simulink model "acc_with_sensor"  (R2021b)
settings: Solver=FixedStepAuto  StartTime=0.0  StopTime=206  FixedStep=0.0005  RelTol=1e-3
InitFcn:
  | G=9.81;
  | m=1660;
  | rw=0.325;
  | Caf=74070;
  | Car=58525;
  | Iz=2778.5;
  | d = 1.502;
  | lf =1.1135;
  | lr =1.5065;
  | L = 2.62;
  | kph2mps=1/3.6;
values from neighbouring files (symbols this model uses):
  Leftdis_PV_switch = 2    [acc_plot_backup.m]
  s_path = [0 1.10508939428 2.2141958029 3.32141571172 4.42705301151 5.53154548532 6.63517443471 7.73808041313 8.84055018688 9.94289959674 11.0453539299 12.1480581097 ... (1001 elements, 1001x1)]    [200_100radius.mat]    (also in LV_Clothoid_S_Turn_path.mat = [0 0.966832089581 1.93621320584 2.90214024471 3.86476766313 ; NEDC_path.mat = [0 0.414605943146 0.832514087334 1.25401518562 1.68216660344; Straight_East_into_curve.mat = [0 1.65770560069 3.32192925577 4.98420060507 6.64484613518 8; acc_plot_backup.m = Station_HV_m)
  X_path = [0 1.10508939428 2.2141958029 3.32141571172 4.42705301151 5.53154548532 6.63517443471 7.73808041313 8.84055018688 9.94289959674 11.0453539299 12.1480581097 ... (1001 elements, 1001x1)]    [200_100radius.mat]    (also in LV_Clothoid_S_Turn_path.mat = [-10 -9.03316791042 -8.06378679416 -7.09785975529 -6.1352323; NEDC_path.mat = [0 0.414605943146 0.832514087334 1.25401518562 1.68216660344; Straight_East_into_curve.mat = [0 1.65770560069 3.32192925577 4.98420060507 6.64484613518 8; acc_plot_backup.m = X_HV_m)
  Y_path = [0 -1.70364610795e-18 -7.41532896709e-18 1.46822109542e-17 4.74557362791e-17 6.12980216762e-17 9.25043977736e-17 1.24088240159e-16 1.5099156923e-16 1.7058517853e-16 1.90629227614e-16 2.09673434424e-16 ... (1001 elements, 1001x1)]    [200_100radius.mat]    (also in LV_Clothoid_S_Turn_path.mat = [0 -8.46153035536e-19 5.07382551045e-18 2.07356032218e-17 3.; NEDC_path.mat = [0 -3.50680326162e-18 -2.14111304971e-18 3.38197671014e-18 3; Straight_East_into_curve.mat = [0 1.29197709199e-18 2.81882429322e-18 3.49020462564e-17 6.7; acc_plot_backup.m = Y_HV_m)
undefined symbols (not defined in the file or in its folder): C_TICK_TIME_S, Cut_in_Secenary_flg, ENUM_ACCSTATE_DISABLED, ENUM_ACCSTATE_OFF, ENUM_ACCSTATE_STANDBY, FALSE, KVDI_ACCLongPressTime_ms, KVDI_ACCMaxActSpeed_kph, KVDI_ACCSetSpdIntial_kph, KVDI_ACCSpdLargeChange_kph, KVDI_LongPressConTime_ms, ONE_FLOAT, ONE_INT, raptor_xcp_function, T, TRUE, UseTTC_switch, ZERO_FLOAT, ZERO_INT
libraries: ADASLibrary x29, simulink x22, Raptor_lib x11, dspstat3 x6, simulink_extras x6, Solver_SF x1, mpclib x1
(part 4 of 9)

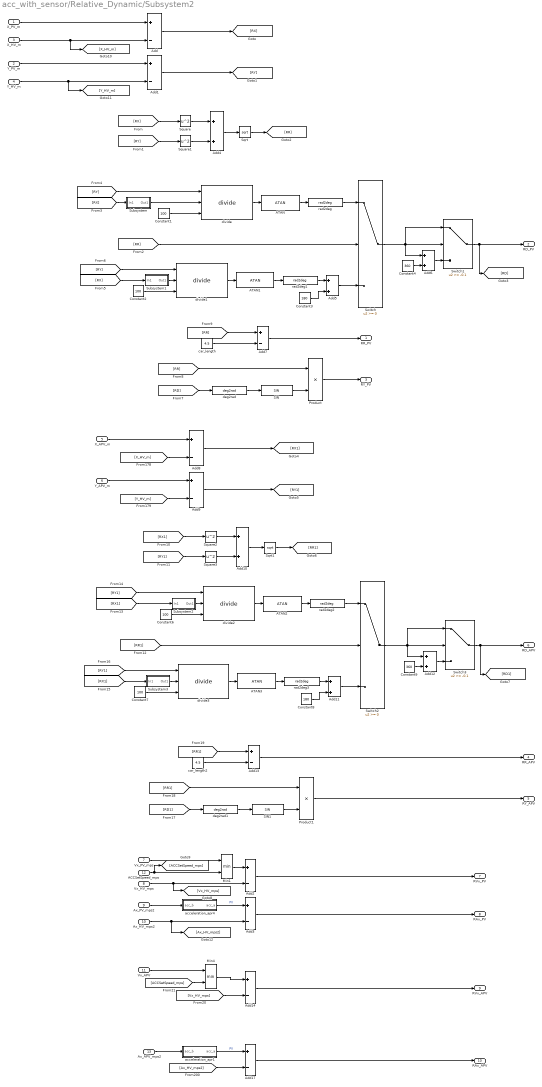
== system acc_with_sensor/Relative_Dynamic/Subsystem2 ==
  X_PV_m : Inport
  Y_PV_m : Inport  Port=2
  X_HV_m : Inport  Port=3
  Y_HV_m : Inport  Port=4
  X_APV_m : Inport  Port=5
  Y_APV_m : Inport  Port=6
  Vx_PV_mps : Inport  Port=7
  Vx_HV_mps : Inport  Port=8
  Ax_PV_mps2 : Inport  Port=9
  Ax_HV_mps2 : Inport  Port=10
  Vx_APV : Inport  Port=11
  ACCSetSpeed_mps : Inport  Port=12
  Ax_APV_mps2 : Inport  Port=13
  ATAN{,1..3} (4 alike) : ADASLibrary/ATAN
      settings: SourceProductName=ADASLibrary
  Add{,1..3,7..9,13..14,17} (10 alike) : Sum  Inputs=+-
  Add{4..6,10..12} (6 alike) : Sum
  Constant{1..2,6..7} (4 alike) : Constant  Value=100  SampleTime=T
  Constant3 : Constant  Value=180  SampleTime=T
  Constant4 : Constant  Value=360  SampleTime=T
  Constant8 : Constant  Value=180  SampleTime=T
  Constant9 : Constant  Value=360  SampleTime=T
  Min1 : MinMax  Inputs=2
  Min4 : MinMax  Inputs=2
  Product : Product
  Product1 : Product
  SIN : ADASLibrary/SIN
      settings: SourceProductName=ADASLibrary
  SIN1 : ADASLibrary/SIN
      settings: SourceProductName=ADASLibrary
  Sqrt : Sqrt  SaturateOnIntegerOverflow=on
  Sqrt1 : Sqrt  SaturateOnIntegerOverflow=on
  Square{,1..3} (4 alike) : Math  Operator=square  SaturateOnIntegerOverflow=on
  Subsystem : Subsystem
  Subsystem1 : Subsystem
  Subsystem2 : Subsystem
  Subsystem3 : Subsystem
  Switch : Switch
  Switch1 : Switch  Threshold=-0.1
  Switch2 : Switch
  Switch3 : Switch  Threshold=-0.1
  acceleration_apr1 : Subsystem
  acceleration_apr4 : Subsystem
  car_length : Constant  Value=4.5  SampleTime=T
  car_length2 : Constant  Value=4.5  SampleTime=T
  deg2rad : ADASLibrary/deg2rad
      settings: SourceProductName=ADASLibrary
  deg2rad1 : ADASLibrary/deg2rad
      settings: SourceProductName=ADASLibrary
  divide{,1..3} (4 alike) : ADASLibrary/divide  Upper_limit=0.001  Lower_limit=-0.001
      settings: SourceProductName=ADASLibrary
  rad2deg{,1..3} (4 alike) : ADASLibrary/rad2deg
      settings: SourceProductName=ADASLibrary
  RR_PV : Outport
  RD_PV : Outport  Port=2
  RY_PV : Outport  Port=3
  RR_APV : Outport  Port=4
  RY_APV : Outport  Port=5
  RD_APV : Outport  Port=6
  RVx_PV : Outport  Port=7
  RAx_PV : Outport  Port=8
  RVx_APV : Outport  Port=9
  RAx_APV : Outport  Port=10
  wires:
  Ax_PV_mps2/1 -> acceleration_apr4/1(acc_b)
  Vx_PV_mps/1 -> Min1/1
  Add14/1 -> RVx_APV/1
  [Vx_HV_mps] -> Add14/2
  Add2/1 -> RVx_PV/1
  Min4/1 -> Add14/1
  acceleration_apr1/1(acc_a) -> Add17/1  "PV"
  Add17/1 -> RAx_APV/1
  acceleration_apr4/1(acc_a) -> Add3/1  "PV"
  Add3/1 -> RAx_PV/1
  Vx_APV/1 -> Min4/1
  Vx_HV_mps/1 -> [Vx_HV_mps], Add2/2
  Ax_APV_mps2/1 -> acceleration_apr1/1(acc_b)
  [Ax_HV_mps2] -> Add17/2
  Ax_HV_mps2/1 -> Add3/2, [Ax_HV_mps2]
  [ACCSetSpeed_mps] -> Min4/2
  X_PV_m/1 -> Add/1
  X_HV_m/1 -> Add/2, [X_HV_m]
  Add1/1 -> [RY]
  Y_HV_m/1 -> Add1/2, [Y_HV_m]
  Y_PV_m/1 -> Add1/1
  Add/1 -> [RX]
  [RX] -> Square/1
  [RY] -> Square1/1
  Square/1 -> Add4/1
  Square1/1 -> Add4/2
  Add4/1 -> Sqrt/1
  Sqrt/1 -> [RR]
  [RR] -> Switch/2
  ATAN/1 -> rad2deg/1
  [RY] -> divide/1
  Constant1/1 -> divide/3
  divide/1 -> ATAN/1
  rad2deg/1 -> Switch/1
  divide1/1 -> ATAN1/1
  Constant2/1 -> divide1/3
  [RX] -> Subsystem1/1(In1)
  [RY] -> divide1/1
  ATAN1/1 -> rad2deg1/1
  rad2deg1/1 -> Add5/1
  Add5/1 -> Switch/3
  Constant3/1 -> Add5/2
  Switch/1 -> Add6/1, Switch1/2, Switch1/1
  Switch1/1 -> [RD], RD_PV/1
  Add6/1 -> Switch1/3
  Constant4/1 -> Add6/2
  [RR] -> Product/1
  [RD] -> deg2rad/1
  deg2rad/1 -> SIN/1
  SIN/1 -> Product/2
  Product/1 -> RY_PV/1
  [RR] -> Add7/1
  Add7/1 -> RR_PV/1
  car_length/1 -> Add7/2
  Add8/1 -> [RX1]
  Y_APV_m/1 -> Add9/1
  [Y_HV_m] -> Add9/2
  Add9/1 -> [RY1]
  [X_HV_m] -> Add8/2
  X_APV_m/1 -> Add8/1
  Sqrt1/1 -> [RR1]
  Add10/1 -> Sqrt1/1
  Square3/1 -> Add10/2
  Square2/1 -> Add10/1
  [RY1] -> Square3/1
  [RX1] -> Square2/1
  Constant9/1 -> Add12/2
  Add12/1 -> Switch3/3
  Switch3/1 -> RD_APV/1, [RD1]
  Switch2/1 -> Switch3/1, Switch3/2, Add12/1
  Constant8/1 -> Add11/2
  Add11/1 -> Switch2/3
  rad2deg3/1 -> Add11/1
  ATAN3/1 -> rad2deg3/1
  [RY1] -> divide3/1
  [RX1] -> Subsystem3/1(In1)
  Constant7/1 -> divide3/3
  divide3/1 -> ATAN3/1
  rad2deg2/1 -> Switch2/1
  divide2/1 -> ATAN2/1
  Constant6/1 -> divide2/3
  [RX1] -> Subsystem2/1(In1)
  [RY1] -> divide2/1
  ATAN2/1 -> rad2deg2/1
  [RR1] -> Switch2/2
  car_length2/1 -> Add13/2
  Add13/1 -> RR_APV/1
  [RR1] -> Add13/1
  SIN1/1 -> Product1/2
  deg2rad1/1 -> SIN1/1
  [RD1] -> deg2rad1/1
  [RR1] -> Product1/1
  Product1/1 -> RY_APV/1
  [RX] -> Subsystem/1(In1)
  Subsystem/1(Out1) -> divide/2
  Subsystem1/1(Out1) -> divide1/2
  Subsystem2/1(Out1) -> divide2/2
  Subsystem3/1(Out1) -> divide3/2
  Min1/1 -> Add2/1
  ACCSetSpeed_mps/1 -> Min1/2, [ACCSetSpeed_mps]

== system acc_with_sensor/Relative_Dynamic/Subsystem5 ==
  OnlyPV_signal : Inport
  RR_PV : Inport  Port=2
  RVx_PV : Inport  Port=3
  RAx_PV : Inport  Port=4
  RR_APV : Inport  Port=5
  RVx_APV : Inport  Port=6
  RAx_APV : Inport  Port=7
  RY_PV : Inport  Port=8
  RY_APV : Inport  Port=9
  In10 : Inport  Port=10
  In11 : Inport  Port=11
  Enable : EnablePort  StatesWhenEnabling=reset
  Abs2 : Abs
  Abs3 : Abs
  MATLAB Function7 : MATLAB Function  TreatAsAtomicUnit=on
  RR : Outport
  RV : Outport  Port=2
  RA : Outport  Port=3
  trig : Outport  Port=4
  wires:
  Abs2/1 -> MATLAB Function7/10(RD_PV)
  Abs3/1 -> MATLAB Function7/11(RD_APV)
  MATLAB Function7/4(trig) -> trig/1
  MATLAB Function7/3(RA) -> RA/1
  OnlyPV_signal/1 -> MATLAB Function7/1(OnlyPV_signal)
  MATLAB Function7/2(RV) -> RV/1
  MATLAB Function7/1(RR) -> RR/1
  RR_PV/1 -> MATLAB Function7/2(RR_PV)
  RR_APV/1 -> MATLAB Function7/3(RR_APV)
  RVx_PV/1 -> MATLAB Function7/4(RVx_PV)
  RVx_APV/1 -> MATLAB Function7/5(RVx_APV)
  RAx_PV/1 -> MATLAB Function7/6(RAx_PV)
  RAx_APV/1 -> MATLAB Function7/7(RAx_APV)
  RY_PV/1 -> MATLAB Function7/8(RY_PV)
  RY_APV/1 -> MATLAB Function7/9(RY_APV)
  In10/1 -> Abs2/1
  In11/1 -> Abs3/1

== system acc_with_sensor/Relative_Dynamic/Subsystem8 ==
  PV_RR : Inport
  APV_RR : Inport  Port=2
  PV_RV : Inport  Port=3
  APV_RV : Inport  Port=4
  PV_RA : Inport  Port=5
  APV_RA : Inport  Port=6
  Constant : Constant  Value=Cut_in_Secenary_flg
  Switch14 : Switch  Criteria=u2 ~= 0
  Switch15 : Switch  Criteria=u2 ~= 0
  Switch7 : Switch  Criteria=u2 ~= 0
  RR_PV : Outport
  RV_PV : Outport  Port=2
  RA_PV : Outport  Port=3
  wires:
  Switch15/1 -> RA_PV/1
  [RR_APV] -> Switch7/1
  [RR_PV] -> Switch7/3
  [RAx_APV] -> Switch15/1
  Switch7/1 -> RR_PV/1
  [RVx_PV] -> Switch14/3
  Switch14/1 -> RV_PV/1
  Constant/1 -> Switch7/2, Switch14/2, Switch15/2
  [RVx_APV] -> Switch14/1
  [RAx_PV] -> Switch15/3
  PV_RR/1 -> [RR_PV]
  APV_RR/1 -> [RR_APV]
  PV_RV/1 -> [RVx_PV]
  APV_RV/1 -> [RVx_APV]
  PV_RA/1 -> [RAx_PV]
  APV_RA/1 -> [RAx_APV]

== system acc_with_sensor/Smooth Switch/Subsystem ==
  TTC : Inport
  Mode : Inport  Port=2
  1-D Lookup Table : Lookup_n-D  NumberOfTableDimensions=1  BreakpointsForDimension1=[0 2 10]  Table=[0.05 0.05 0.5]  InternalRulePriority=Speed  RndMeth=Simplest  InputSameDT=on
  Constant1 : Constant  Value=0.5
  Constant2 : Constant
  Constant3 : Constant  Value=0.01
  Switch : Switch  Criteria=u2 ~= 0
  tau : Outport
  wires:
  Constant1/1 -> Switch/1
  Switch/1 -> tau/1
  Mode/1 -> Switch/2
  TTC/1 -> 1-D Lookup Table/1
  1-D Lookup Table/1 -> Switch/3

== system acc_with_sensor/Smooth Switch1/Smooth_Switch1 ==
  In1 : Inport
  Add : Sum
  Add1 : Sum  Inputs=+-
  Constant : Constant  Value=T/tau
  Constant1 : Constant
  Product : Product
  Product1 : Product
  Unit Delay : UnitDelay  InitialCondition=IC  SampleTime=T  HasFrameUpgradeWarning=on
  Out1 : Outport
  wires:
  Constant1/1 -> Add1/1
  Constant/1 -> Add1/2, Product1/2
  Add1/1 -> Product/1
  In1/1 -> Product1/1
  Product/1 -> Add/2
  Unit Delay/1 -> Product/2, Out1/1
  Add/1 -> Unit Delay/1
  Product1/1 -> Add/1

== system acc_with_sensor/Smooth Switch4/Subsystem ==
  Constant1 : Constant  Value=0.5
  tau : Outport
  wires:
  Constant1/1 -> tau/1

== system acc_with_sensor/Subsystem/cut_off5 ==
  sign : Inport
  in : Inport  Port=2
  Delay : Delay  DelayLength=1  InitialConditionSource=Input port
      settings: InputPortMap=u0,p4
  Switch16 : Switch  Criteria=u2 ~= 0
  Out : Outport  VectorParamsAs1DForOutWhenUnconnected=off
  wires:
  in/1 -> Delay/2, Switch16/3
  sign/1 -> Switch16/2
  Switch16/1 -> Out/1, Delay/1
  Delay/1 -> Switch16/1

== system acc_with_sensor/Subsystem17/rolling_avg1 ==
  note: new_average = [ (sample_interval)/(sample_interval + time_constant) ] * (new_value - old_ave) + old_ave
  note: - (FK_TMR/TC)
      |                                    f  =  1  -  e
      |
      |       Where "f" is called the filter constant in the difference equation:
      |
      |                    new_average = f * new_value + (1 - f) * old_average
  note: Using the first two terms of the series expansion:
      |
      |                     x                     x2
      |                                e   =  1  +  x  +  --  + ......
      |                                           2!
      |
      |       Simplifying, the exponential "f" becomes:
      |
      |                  - (FK_TMR/TC)              1
      |           f  =  1  -  e                    =  1  -  -------------  =  . . .
      |                                                    (FK_TMR/TC)
      |                           e
      |
      |                              1                      1
      |          f  =  1  -  ---------------------------------  =    ------------------- .
      |                                  1 + (FK_TMR / TC)       1 + (TC / FK_TMR)
  new_value : Inport
  old_ave : Inport  Port=2
  delta_t : Inport  Port=3
  tc : Inport  Port=4
  Divide : Product  Inputs=*/
  IC : UnitDelay  Tag=struct('comment',struct('text','','placement',1),'logdata',struct('maxnumvals',inf,'plotchannels',[],'stepsize',0,'downsampling',1,'loggingmode',3,'channels',1),'output',struct('width',1,'name','$S_$B','unit','','type','Int16','offset',0,'max',NaN,'min',NaN,'freeze',1,'lsb',1,'arb',0,'class','default','address','','description','','autoscalingmode',1,'lowerheadroom',1,'upperheadroom',1,'headroomunit','bit','checkmin',0,'checkmax',0,'show',0,'initial','2'),'state',0,'dt','-1','date',731455.586925799)  InitialCondition=1  SampleTime=T  HasFrameUpgradeWarning=on
  Interval Test : simulink/Logic and Bit Operations/Interval Test  IntervalClosedRight=on  uplimit=0.00001  IntervalClosedLeft=on  lowlimit=-0.00001  OutDataTypeStr=boolean
  Logical Operator : Logic  Operator=NOT  AllPortsSameDT=off  OutDataTypeStr=boolean
  Product_tmp1 : Product  Tag=struct('comment',struct('text','','placement',1),'logdata',struct('maxnumvals',inf,'plotchannels',[],'stepsize',0,'downsampling',1,'loggingmode',3,'channels',1),'output',struct('width',1,'name','$S_$B','unit','','type','Int32Bin15','offset',0,'max',65535,'min',-65536,'freeze',1,'lsb',2^-15,'arb',0,'class','default','address','','description','','autoscalingmode',1,'lowerheadroom',1,'upperheadroom',1,'headroomunit','bit','checkmin',0,'checkmax',0,'show',0),'inputs','**','exceptionhandling',1,'date',731455.58640515)  Inputs=**  InputSameDT=on  RndMeth=Zero  OutDataTypeStr=Inherit: Same as first input
  Sum : Sum  Tag=struct('comment',struct('text','','placement',1),'logdata',struct('maxnumvals',inf,'plotchannels',[],'stepsize',0,'downsampling',1,'loggingmode',3,'channels',1),'output',struct('width',1,'name','$S_$B','unit','','type','Int32Bin15','offset',0,'max',65535,'min',-65536,'freeze',1,'lsb',2^-15,'arb',0,'class','default','address','','description','','autoscalingmode',1,'lowerheadroom',1,'upperheadroom',1,'headroomunit','bit','checkmin',0,'checkmax',0,'show',0),'inputs','-+','date',731455.586330463)  Inputs=-+  InputSameDT=on  OutDataTypeStr=Inherit: Same as first input
  Sum1 : Sum  Tag=struct('comment',struct('text','','placement',1),'logdata',struct('maxnumvals',inf,'plotchannels',[],'stepsize',0,'downsampling',1,'loggingmode',3,'channels',1),'output',struct('width',1,'name','$S_$B','unit','','type','Int32Bin15','offset',0,'max',65535,'min',-65536,'freeze',1,'lsb',2^-15,'arb',0,'class','default','address','','description','','autoscalingmode',1,'lowerheadroom',1,'upperheadroom',1,'headroomunit','bit','checkmin',0,'checkmax',0,'show',0),'inputs','++','date',731455.58628235)  InputSameDT=on  OutDataTypeStr=Inherit: Same as first input
  Sum2 : Sum  Tag=struct('comment',struct('text','','placement',1),'logdata',struct('maxnumvals',inf,'plotchannels',[],'stepsize',0,'downsampling',1,'loggingmode',3,'channels',1),'output',struct('width',1,'name','$S_$B','unit','','type','Int32Bin15','offset',0,'max',65535,'min',-65536,'freeze',1,'lsb',2^-15,'arb',0,'class','default','address','','description','','autoscalingmode',1,'lowerheadroom',1,'upperheadroom',1,'headroomunit','bit','checkmin',0,'checkmax',0,'show',0),'inputs','++','date',731455.586506424)  InputSameDT=on  OutDataTypeStr=Inherit: Same as first input
  Switch : Switch  Criteria=u2 ~= 0
  Switch1 : Switch  Tag=struct('comment',struct('text','','placement',1),'logdata',struct('maxnumvals',inf,'plotchannels',[],'stepsize',0,'downsampling',1,'loggingmode',3,'channels',1),'output',struct('width',1,'name','$S_$B','unit','','type','Int32Bin15','offset',0,'max',65535,'min',-65536,'freeze',1,'lsb',2^-15,'arb',0,'class','default','address','','description','','autoscalingmode',1,'lowerheadroom',1,'upperheadroom',1,'headroomunit','bit','checkmin',0,'checkmax',0,'show',0),'threshold',struct('width',1,'name','$S_$B_threshold','unit','','type','Int16','offset',0,'max',NaN,'min',NaN,'freeze',1,'lsb',1,'arb',0,'class','default','address','','description','','value','1','scalar',0),'date',731455.58657044)  Threshold=0.5  InputSameDT=on
  zero : Constant  Tag=struct('comment',struct('text','','placement',1),'output',struct('width',1,'name','$S_$B','unit','','type','Int16','offset',0,'max',NaN,'min',NaN,'freeze',1,'lsb',1,'arb',0,'class','default','address','','description','','value','0','tolerance',1,'show',0),'date',731455.58675544)  Value=0  OutDataTypeStr=Inherit: Inherit via back propagation
  zero1 : Constant  Tag=struct('comment',struct('text','','placement',1),'output',struct('width',1,'name','$S_$B','unit','','type','Int16','offset',0,'max',NaN,'min',NaN,'freeze',1,'lsb',1,'arb',0,'class','default','address','','description','','value','0','tolerance',1,'show',0),'date',731455.58675544)  Value=0  OutDataTypeStr=Inherit: Inherit via back propagation
  new_ave : Outport
  wires:
  Switch/1 -> Sum2/2
  Product_tmp1/1 -> Divide/1
  [new_value] -> Switch1/1
  Sum2/1 -> Switch1/3  "new_ave"
  new_value/1 -> [new_value], Sum/2  "new_value"
  Switch1/1 -> new_ave/1  "new_ave"
  Sum/1 -> Product_tmp1/1
  tc/1 -> Sum1/2
  delta_t/1 -> Sum1/1, Product_tmp1/2  "delta_t"
  zero/1 -> IC/1
  old_ave/1 -> Sum/1, Sum2/1  "old_ave"
  Sum1/1 -> Interval Test/1, Divide/2
  zero1/1 -> Switch/3
  Interval Test/1 -> Logical Operator/1
  Divide/1 -> Switch/1
  Logical Operator/1 -> Switch/2
  IC/1 -> Switch1/2

== system acc_with_sensor/Subsystem2/Smooth_Switch1 ==
  In1 : Inport
  Add : Sum
  Add1 : Sum  Inputs=+-
  Constant : Constant  Value=T/tau
  Constant1 : Constant
  Product : Product
  Product1 : Product
  Unit Delay : UnitDelay  InitialCondition=IC  SampleTime=T  HasFrameUpgradeWarning=on
  Out1 : Outport
  wires:
  Constant1/1 -> Add1/1
  Constant/1 -> Add1/2, Product1/2
  Add1/1 -> Product/1
  In1/1 -> Product1/1
  Product/1 -> Add/2
  Unit Delay/1 -> Product/2, Out1/1
  Add/1 -> Unit Delay/1
  Product1/1 -> Add/1

== system acc_with_sensor/Subsystem2/Smooth_Switch2 ==
  In1 : Inport
  Add : Sum
  Add1 : Sum  Inputs=+-
  Constant : Constant  Value=T/tau
  Constant1 : Constant
  Product : Product
  Product1 : Product
  Unit Delay : UnitDelay  InitialCondition=IC  SampleTime=T  HasFrameUpgradeWarning=on
  Out1 : Outport
  wires:
  Product1/1 -> Add/1
  Add/1 -> Unit Delay/1
  Unit Delay/1 -> Out1/1, Product/2
  Product/1 -> Add/2
  In1/1 -> Product1/1
  Add1/1 -> Product/1
  Constant/1 -> Product1/2, Add1/2
  Constant1/1 -> Add1/1

== system acc_with_sensor/Subsystem2/Subsystem ==
  new_value : Inport
  Constant83 : Constant  Value=0.3
  Constant84 : Constant  Value=0.1
  Delay11 : Delay  DelayLength=1  SampleTime=T
  rolling_avg1 : Subsystem
  new_ave : Outport
  wires:
  Constant84/1 -> rolling_avg1/3(delta_t)  "T"
  rolling_avg1/1(new_ave) -> Delay11/1, new_ave/1
  Delay11/1 -> rolling_avg1/2(old_ave)
  Constant83/1 -> rolling_avg1/4(tc)
  new_value/1 -> rolling_avg1/1(new_value)

== system acc_with_sensor/Subsystem2/Subsystem1 ==
  new_value : Inport
  Constant83 : Constant  Value=0.3
  Constant84 : Constant  Value=0.1
  Delay11 : Delay  DelayLength=1  SampleTime=T
  rolling_avg1 : Subsystem
  new_ave : Outport
  wires:
  new_value/1 -> rolling_avg1/1(new_value)
  Constant83/1 -> rolling_avg1/4(tc)
  Delay11/1 -> rolling_avg1/2(old_ave)
  rolling_avg1/1(new_ave) -> new_ave/1, Delay11/1
  Constant84/1 -> rolling_avg1/3(delta_t)  "T"

== system acc_with_sensor/Subsystem22/Subsystem ==
  In1 : Inport
  Abs : Abs
  Constant : Constant  Value=0
  Switch : Switch  Criteria=u2 > Threshold  Threshold=1
  Out1 : Outport
  wires:
  In1/1 -> Switch/1, Abs/1
  Abs/1 -> Switch/2
  Constant/1 -> Switch/3
  Switch/1 -> Out1/1

== system acc_with_sensor/Subsystem22/cmd_limiter1 ==
  ax_cmd : Inport
  Constant : Constant  Value=0.1  SampleTime=T
  Constant1 : Constant  Value=2.5  SampleTime=T
  Constant2 : Constant  Value=-2.5  SampleTime=T
  Constant3 : Constant  Value=2  SampleTime=T
  Constant4 : Constant  Value=-2  SampleTime=T
  Limit : ADASLibrary/Limit  SystemSampleTime=-1  VariantActivationTime=update diagram  Latency=0  AutoFrameSizeCalculation=off
      settings: SourceProductName=ADASLibrary
  rate_limit : Subsystem
  ax_cmd1 : Outport
  wires:
  rate_limit/1(ax_cmd1) -> ax_cmd1/1
  Constant/1 -> rate_limit/2(Sample_Time)
  ax_cmd/1 -> Limit/1
  Constant1/1 -> rate_limit/3(ratelimt_incps)
  Constant2/1 -> rate_limit/4(ratelimt_decps)
  Limit/1 -> rate_limit/1(input_raw)
  Constant3/1 -> Limit/2
  Constant4/1 -> Limit/3

== system acc_with_sensor/Subsystem22/cmd_limiter2 ==
  ax_cmd : Inport
  Constant : Constant  Value=0.1  SampleTime=T
  Constant1 : Constant  Value=2.5  SampleTime=T
  Constant2 : Constant  Value=-2.5  SampleTime=T
  Constant3 : Constant  Value=2  SampleTime=T
  Constant4 : Constant  Value=-2  SampleTime=T
  Limit : ADASLibrary/Limit  SystemSampleTime=-1  VariantActivationTime=update diagram  Latency=0  AutoFrameSizeCalculation=off
      settings: SourceProductName=ADASLibrary
  rate_limit : Subsystem
  ax_cmd1 : Outport
  wires:
  Constant4/1 -> Limit/3
  Constant3/1 -> Limit/2
  Limit/1 -> rate_limit/1(input_raw)
  Constant2/1 -> rate_limit/4(ratelimt_decps)
  Constant1/1 -> rate_limit/3(ratelimt_incps)
  ax_cmd/1 -> Limit/1
  Constant/1 -> rate_limit/2(Sample_Time)
  rate_limit/1(ax_cmd1) -> ax_cmd1/1

== system acc_with_sensor/Subsystem4/rolling_avg1 ==
  note: Using the first two terms of the series expansion:
      |
      |                     x                     x2
      |                                e   =  1  +  x  +  --  + ......
      |                                           2!
      |
      |       Simplifying, the exponential "f" becomes:
      |
      |                  - (FK_TMR/TC)              1
      |           f  =  1  -  e                    =  1  -  -------------  =  . . .
      |                                                    (FK_TMR/TC)
      |                           e
      |
      |                              1                      1
      |          f  =  1  -  ---------------------------------  =    ------------------- .
      |                                  1 + (FK_TMR / TC)       1 + (TC / FK_TMR)
  note: - (FK_TMR/TC)
      |                                    f  =  1  -  e
      |
      |       Where "f" is called the filter constant in the difference equation:
      |
      |                    new_average = f * new_value + (1 - f) * old_average
  note: new_average = [ (sample_interval)/(sample_interval + time_constant) ] * (new_value - old_ave) + old_ave
  new_value : Inport
  old_ave : Inport  Port=2
  delta_t : Inport  Port=3
  tc : Inport  Port=4
  Divide : Product  Inputs=*/
  IC : UnitDelay  Tag=struct('comment',struct('text','','placement',1),'logdata',struct('maxnumvals',inf,'plotchannels',[],'stepsize',0,'downsampling',1,'loggingmode',3,'channels',1),'output',struct('width',1,'name','$S_$B','unit','','type','Int16','offset',0,'max',NaN,'min',NaN,'freeze',1,'lsb',1,'arb',0,'class','default','address','','description','','autoscalingmode',1,'lowerheadroom',1,'upperheadroom',1,'headroomunit','bit','checkmin',0,'checkmax',0,'show',0,'initial','2'),'state',0,'dt','-1','date',731455.586925799)  InitialCondition=1  SampleTime=T  HasFrameUpgradeWarning=on
  Interval Test : simulink/Logic and Bit Operations/Interval Test  IntervalClosedRight=on  uplimit=0.00001  IntervalClosedLeft=on  lowlimit=-0.00001  OutDataTypeStr=boolean
  Logical Operator : Logic  Operator=NOT  AllPortsSameDT=off  OutDataTypeStr=boolean
  Product_tmp1 : Product  Tag=struct('comment',struct('text','','placement',1),'logdata',struct('maxnumvals',inf,'plotchannels',[],'stepsize',0,'downsampling',1,'loggingmode',3,'channels',1),'output',struct('width',1,'name','$S_$B','unit','','type','Int32Bin15','offset',0,'max',65535,'min',-65536,'freeze',1,'lsb',2^-15,'arb',0,'class','default','address','','description','','autoscalingmode',1,'lowerheadroom',1,'upperheadroom',1,'headroomunit','bit','checkmin',0,'checkmax',0,'show',0),'inputs','**','exceptionhandling',1,'date',731455.58640515)  Inputs=**  InputSameDT=on  RndMeth=Zero  OutDataTypeStr=Inherit: Same as first input
  Sum : Sum  Tag=struct('comment',struct('text','','placement',1),'logdata',struct('maxnumvals',inf,'plotchannels',[],'stepsize',0,'downsampling',1,'loggingmode',3,'channels',1),'output',struct('width',1,'name','$S_$B','unit','','type','Int32Bin15','offset',0,'max',65535,'min',-65536,'freeze',1,'lsb',2^-15,'arb',0,'class','default','address','','description','','autoscalingmode',1,'lowerheadroom',1,'upperheadroom',1,'headroomunit','bit','checkmin',0,'checkmax',0,'show',0),'inputs','-+','date',731455.586330463)  Inputs=-+  InputSameDT=on  OutDataTypeStr=Inherit: Same as first input
  Sum1 : Sum  Tag=struct('comment',struct('text','','placement',1),'logdata',struct('maxnumvals',inf,'plotchannels',[],'stepsize',0,'downsampling',1,'loggingmode',3,'channels',1),'output',struct('width',1,'name','$S_$B','unit','','type','Int32Bin15','offset',0,'max',65535,'min',-65536,'freeze',1,'lsb',2^-15,'arb',0,'class','default','address','','description','','autoscalingmode',1,'lowerheadroom',1,'upperheadroom',1,'headroomunit','bit','checkmin',0,'checkmax',0,'show',0),'inputs','++','date',731455.58628235)  InputSameDT=on  OutDataTypeStr=Inherit: Same as first input
  Sum2 : Sum  Tag=struct('comment',struct('text','','placement',1),'logdata',struct('maxnumvals',inf,'plotchannels',[],'stepsize',0,'downsampling',1,'loggingmode',3,'channels',1),'output',struct('width',1,'name','$S_$B','unit','','type','Int32Bin15','offset',0,'max',65535,'min',-65536,'freeze',1,'lsb',2^-15,'arb',0,'class','default','address','','description','','autoscalingmode',1,'lowerheadroom',1,'upperheadroom',1,'headroomunit','bit','checkmin',0,'checkmax',0,'show',0),'inputs','++','date',731455.586506424)  InputSameDT=on  OutDataTypeStr=Inherit: Same as first input
  Switch : Switch  Criteria=u2 ~= 0
  Switch1 : Switch  Tag=struct('comment',struct('text','','placement',1),'logdata',struct('maxnumvals',inf,'plotchannels',[],'stepsize',0,'downsampling',1,'loggingmode',3,'channels',1),'output',struct('width',1,'name','$S_$B','unit','','type','Int32Bin15','offset',0,'max',65535,'min',-65536,'freeze',1,'lsb',2^-15,'arb',0,'class','default','address','','description','','autoscalingmode',1,'lowerheadroom',1,'upperheadroom',1,'headroomunit','bit','checkmin',0,'checkmax',0,'show',0),'threshold',struct('width',1,'name','$S_$B_threshold','unit','','type','Int16','offset',0,'max',NaN,'min',NaN,'freeze',1,'lsb',1,'arb',0,'class','default','address','','description','','value','1','scalar',0),'date',731455.58657044)  Threshold=0.5  InputSameDT=on
  zero : Constant  Tag=struct('comment',struct('text','','placement',1),'output',struct('width',1,'name','$S_$B','unit','','type','Int16','offset',0,'max',NaN,'min',NaN,'freeze',1,'lsb',1,'arb',0,'class','default','address','','description','','value','0','tolerance',1,'show',0),'date',731455.58675544)  Value=0  OutDataTypeStr=Inherit: Inherit via back propagation
  zero1 : Constant  Tag=struct('comment',struct('text','','placement',1),'output',struct('width',1,'name','$S_$B','unit','','type','Int16','offset',0,'max',NaN,'min',NaN,'freeze',1,'lsb',1,'arb',0,'class','default','address','','description','','value','0','tolerance',1,'show',0),'date',731455.58675544)  Value=0  OutDataTypeStr=Inherit: Inherit via back propagation
  new_ave : Outport
  wires:
  IC/1 -> Switch1/2
  Logical Operator/1 -> Switch/2
  Divide/1 -> Switch/1
  Interval Test/1 -> Logical Operator/1
  zero1/1 -> Switch/3
  Sum1/1 -> Divide/2, Interval Test/1
  old_ave/1 -> Sum2/1, Sum/1  "old_ave"
  zero/1 -> IC/1
  delta_t/1 -> Product_tmp1/2, Sum1/1  "delta_t"
  tc/1 -> Sum1/2
  Sum/1 -> Product_tmp1/1
  Switch1/1 -> new_ave/1  "new_ave"
  new_value/1 -> Sum/2, [new_value]  "new_value"
  Sum2/1 -> Switch1/3  "new_ave"
  [new_value] -> Switch1/1
  Product_tmp1/1 -> Divide/1
  Switch/1 -> Sum2/2

== system acc_with_sensor/Subsystem5/Lat_selector1 ==
  Vx_HV_mps : Inport
  Steer_Dynamic_deg : Inport  Port=2
  Steer_Kinematic_deg : Inport  Port=3
  Constant30 : Constant  Value=35  SampleTime=T
  Constant32 : Constant  Value=30  SampleTime=T
  Gain31 : Gain  Gain=3.6
  Latch : Subsystem
  Relational Operator : RelationalOperator  OutDataTypeStr=boolean  RndMeth=Simplest
  Relational Operator1 : RelationalOperator  Operator=<=  OutDataTypeStr=boolean  RndMeth=Simplest
  Smooth Switch1 : Subsystem
  Subsystem : Subsystem
  new_ave : Outport
  wires:
  Relational Operator1/1 -> Latch/2(reset)
  Gain31/1 -> Relational Operator/1, Relational Operator1/1  "kph"
  Smooth Switch1/1(ax_cmd) -> Subsystem/1(new_value)
  Relational Operator/1 -> Latch/1(set)
  [Steer_Kinematic_deg] -> Smooth Switch1/3(Kinematic_cmd)
  Constant32/1 -> Relational Operator1/2
  [Steer_Dynamic_deg] -> Smooth Switch1/1(Dynamic_cmd)
  Latch/1(latched) -> Smooth Switch1/2(Mode)
  Constant30/1 -> Relational Operator/2
  Vx_HV_mps/1 -> Gain31/1
  Steer_Dynamic_deg/1 -> [Steer_Dynamic_deg]
  Steer_Kinematic_deg/1 -> [Steer_Kinematic_deg]
  Subsystem/1(new_ave) -> new_ave/1

== system acc_with_sensor/Subsystem5/Latch ==
  set : Inport
  reset : Inport  Port=2
  Delay : Delay  DelayLength=1
  Logical Operator3 : Logic  AllPortsSameDT=off  OutDataTypeStr=boolean
  Logical Operator4 : Logic  Operator=NOT  AllPortsSameDT=off  OutDataTypeStr=boolean
  Switch : Switch  Criteria=u2 ~= 0
  Switch1 : Switch  Criteria=u2 ~= 0
  latched : Outport
  wires:
  Delay/1 -> Switch1/3
  Logical Operator4/1 -> Logical Operator3/2, Switch1/1
  Logical Operator3/1 -> Switch/2
  reset/1 -> Logical Operator4/1, Switch1/2
  Switch/1 -> Delay/1, latched/1
  set/1 -> Switch/1, Logical Operator3/1
  Switch1/1 -> Switch/3

== system acc_with_sensor/Subsystem5/MPC_Dynematc1 ==
  Yref : Inport
  Vx_HV_mps : Inport  Port=2
  Steer_SW_deg : Inport  Port=3
  Ax : Inport  Port=4
  LaneAvail_flg : Inport  Port=5
  Enable : EnablePort  StatesWhenEnabling=reset
  1-D Lookup Table2 : Lookup_n-D  NumberOfTableDimensions=1  BreakpointsForDimension1=[0 10 35 40]/3.6  Table=[0.25 0.25 0.025 0.025]  InternalRulePriority=Speed  RndMeth=Simplest  InputSameDT=on
  Constant : Constant  Value=720  SampleTime=T
  Constant1 : Constant  Value=-720  SampleTime=T
  Gain1 : Gain  Gain=20
  Gain4 : Gain  Gain=pi/180
  Gain6 : Gain  Gain=1/20
  Kinematuc_MPC : MATLAB Function  TreatAsAtomicUnit=on
  Limit : ADASLibrary/Limit  SystemSampleTime=-1  VariantActivationTime=update diagram  Latency=0  AutoFrameSizeCalculation=off
      settings: SourceProductName=ADASLibrary
  R selector : Subsystem
  Radians to Degrees3 : simulink_extras/Transformations/Radians to Degrees
  raptor_adjustment3 : Raptor_lib/Data Storage/raptor_adjustment  Commented=on  paramName='R_K'  nameSource=Parameter  initValue=0.5  dataType=double  storage=Calibration  calDispType=Number  calEnum={'False', 'True'}  calGain=1.0  calOffset=0.0  calMax=inf  calMin=-inf  calFormat='-1'  calUnit=''  calHelp=''  calAccess=1  calFunction=raptor_xcp_function(gcb)  calDispHeaders=off  calColHeaders={'Col1' 'Col2' 'Col3'}  calRowHeaders={'Row1' 'Row2' 'Row3'}
      settings: SourceProductName=Raptor
  Kinematic : Outport
  wires:
  Kinematuc_MPC/1(u_K) -> Radians to Degrees3/1
  Gain4/1 -> Kinematuc_MPC/5(steer_angle_K)
  R selector/1(R) -> Kinematuc_MPC/4(Rs_K)
  1-D Lookup Table2/1 -> Kinematuc_MPC/3(Qs_K)
  Yref/1 -> Kinematuc_MPC/2(Yref_K)
  Gain6/1 -> Gain4/1  "deg"
  Radians to Degrees3/1 -> Gain1/1
  Gain1/1 -> Limit/1  "deg"
  Steer_SW_deg/1 -> Gain6/1
  Constant/1 -> Limit/2
  Constant1/1 -> Limit/3
  Limit/1 -> Kinematic/1
  [Vx_HV_mps] -> 1-D Lookup Table2/1
  [Vx_HV_mps] -> R selector/2(vx)
  LaneAvail_flg/1 -> R selector/1(LaneAvail_fig)
  Vx_HV_mps/1 -> [Vx_HV_mps], Kinematuc_MPC/1(vx_K)

== system acc_with_sensor/Subsystem5/MPC_Dynematc2 ==
  Yref : Inport
  Vx_HV_mps : Inport  Port=2
  Steer_SW_deg : Inport  Port=3
  yaw_rate : Inport  Port=4
  Vy : Inport  Port=5
  Ax : Inport  Port=6
  LaneAvail_flg : Inport  Port=7
  Enable : EnablePort  StatesWhenEnabling=reset
  1-D Lookup Table1 : Lookup_n-D  NumberOfTableDimensions=1  BreakpointsForDimension1=[35 40 70 80]/3.6  Table=[0.01 0.01 0.0025 0.0025]  InternalRulePriority=Speed  RndMeth=Simplest  InputSameDT=on
  Constant : Constant  Value=720  SampleTime=T
  Constant1 : Constant  Value=-720  SampleTime=T
  Gain1 : Gain  Gain=20
  Gain4 : Gain  Gain=pi/180
  Gain6 : Gain  Gain=1/20
  Limit : ADASLibrary/Limit  SystemSampleTime=-1  VariantActivationTime=update diagram  Latency=0  AutoFrameSizeCalculation=off
      settings: SourceProductName=ADASLibrary
  MATLAB Function4 : MATLAB Function  TreatAsAtomicUnit=on
  R selector1 : Subsystem
  Radians to Degrees3 : simulink_extras/Transformations/Radians to Degrees
  raptor_adjustment1 : Raptor_lib/Data Storage/raptor_adjustment  Commented=on  paramName='R_D'  nameSource=Parameter  initValue=0.5  dataType=double  storage=Calibration  calDispType=Number  calEnum={'False', 'True'}  calGain=1.0  calOffset=0.0  calMax=inf  calMin=-inf  calFormat='-1'  calUnit=''  calHelp=''  calAccess=1  calFunction=raptor_xcp_function(gcb)  calDispHeaders=off  calColHeaders={'Col1' 'Col2' 'Col3'}  calRowHeaders={'Row1' 'Row2' 'Row3'}
      settings: SourceProductName=Raptor
  Kinematic : Outport
  wires:
  Limit/1 -> Kinematic/1
  Constant1/1 -> Limit/3
  Constant/1 -> Limit/2
  Steer_SW_deg/1 -> Gain6/1
  Gain1/1 -> Limit/1  "deg"
  Radians to Degrees3/1 -> Gain1/1
  Gain6/1 -> Gain4/1  "deg"
  Yref/1 -> MATLAB Function4/2(Yref_D)
  1-D Lookup Table1/1 -> MATLAB Function4/3(Qs_D)
  R selector1/1(R_D) -> MATLAB Function4/4(Rs_D)
  Gain4/1 -> MATLAB Function4/5(steer_angle_D)
  yaw_rate/1 -> MATLAB Function4/6(yaw_rate_D)
  Vy/1 -> MATLAB Function4/7(Vy_D)
  MATLAB Function4/1(u_D) -> Radians to Degrees3/1
  [Vx_HV_mps] -> 1-D Lookup Table1/1
  LaneAvail_flg/1 -> R selector1/1(LaneAvail_flg)
  [Vx_HV_mps] -> R selector1/2(vx)
  Vx_HV_mps/1 -> [Vx_HV_mps], MATLAB Function4/1(Vx_D)

== system acc_with_sensor/Subsystem8/Subsystem ==
  In1 : Inport
  Abs : Abs
  Constant : Constant  Value=0
  Switch : Switch  Criteria=u2 > Threshold  Threshold=1
  Out1 : Outport
  wires:
  In1/1 -> Switch/1, Abs/1
  Abs/1 -> Switch/2
  Constant/1 -> Switch/3
  Switch/1 -> Out1/1

== system acc_with_sensor/Subsystem8/cmd_limiter1 ==
  ax_cmd : Inport
  Constant : Constant  Value=0.1  SampleTime=T
  Constant1 : Constant  Value=2.5  SampleTime=T
  Constant2 : Constant  Value=-2.5  SampleTime=T
  Constant3 : Constant  Value=2  SampleTime=T
  Constant4 : Constant  Value=-2  SampleTime=T
  Limit : ADASLibrary/Limit  SystemSampleTime=-1  VariantActivationTime=update diagram  Latency=0  AutoFrameSizeCalculation=off
      settings: SourceProductName=ADASLibrary
  rate_limit : Subsystem
  ax_cmd1 : Outport
  wires:
  rate_limit/1(ax_cmd1) -> ax_cmd1/1
  Constant/1 -> rate_limit/2(Sample_Time)
  ax_cmd/1 -> Limit/1
  Constant1/1 -> rate_limit/3(ratelimt_incps)
  Constant2/1 -> rate_limit/4(ratelimt_decps)
  Limit/1 -> rate_limit/1(input_raw)
  Constant3/1 -> Limit/2
  Constant4/1 -> Limit/3

== system acc_with_sensor/Subsystem8/cmd_limiter2 ==
  ax_cmd : Inport
  Constant : Constant  Value=0.1  SampleTime=T
  Constant1 : Constant  Value=2.5  SampleTime=T
  Constant2 : Constant  Value=-2.5  SampleTime=T
  Constant3 : Constant  Value=2  SampleTime=T
  Constant4 : Constant  Value=-2  SampleTime=T
  Limit : ADASLibrary/Limit  SystemSampleTime=-1  VariantActivationTime=update diagram  Latency=0  AutoFrameSizeCalculation=off
      settings: SourceProductName=ADASLibrary
  rate_limit : Subsystem
  ax_cmd1 : Outport
  wires:
  Constant4/1 -> Limit/3
  Constant3/1 -> Limit/2
  Limit/1 -> rate_limit/1(input_raw)
  Constant2/1 -> rate_limit/4(ratelimt_decps)
  Constant1/1 -> rate_limit/3(ratelimt_incps)
  ax_cmd/1 -> Limit/1
  Constant/1 -> rate_limit/2(Sample_Time)
  rate_limit/1(ax_cmd1) -> ax_cmd1/1

== system acc_with_sensor/Subsystem8/rate_limit ==
  input_raw : Inport
  Sample_Time : Inport  Port=2
  ratelimt_incps : Inport  Port=3
  ratelimt_decps : Inport  Port=4
  Add : Sum  Inputs=+-
  Add1 : Sum
  Constant : Constant  Value=0  SampleTime=T
  Max : MinMax  Function=max  Inputs=2
  Max1 : MinMax  Inputs=2
  Max2 : MinMax  Function=max  Inputs=2
  Max3 : MinMax  Inputs=2
  Product : Product
  Product1 : Product
  Unit Delay : UnitDelay  SampleTime=T  HasFrameUpgradeWarning=on
  ax_cmd1 : Outport
  wires:
  Product1/1 -> Max2/1
  Product/1 -> Max3/2
  Sample_Time/1 -> Product/1, Product1/2
  ratelimt_incps/1 -> Product1/1
  ratelimt_decps/1 -> Product/2
  Constant/1 -> Max2/2, Max3/1
  Max3/1 -> [Dec]
  Max2/1 -> [Inc]
  Unit Delay/1 -> Add1/2, Add/2
  Add1/1 -> ax_cmd1/1, Unit Delay/1
  Max1/1 -> Add1/1
  [Dec] -> Max/2
  [Inc] -> Max1/1
  Max/1 -> Max1/2
  Add/1 -> Max/1
  input_raw/1 -> Add/1

== system acc_with_sensor/V_rel Estimation/Kalman filter ==
  cut_in_flg : Inport
  Jerk : Inport  Port=2
  S_rel : Inport  Port=3
  initial_value : Inport  Port=4
  Constant : Constant  Value=200  OutDataTypeStr=double
  Constant1 : Constant  Value=0.01  OutDataTypeStr=double
  Delay : Delay  DelayLength=1  InitialCondition=[1 0 0;0 1 0;0 0 1]  SampleTime=T
  Delay1 : Delay  DelayLength=1  InitialConditionSource=Input port  InitialCondition=[1;1;1]  ExternalReset=Rising  SampleTime=T
      settings: InputPortMap=u0,r5,p4
  Demux3 : Demux  Outputs=[1 1 1]
      settings: DisplayOption=none
  MATLAB Function2 : MATLAB Function  TreatAsAtomicUnit=on
  measurement update : MATLAB Function  TreatAsAtomicUnit=on
  time update : MATLAB Function  TreatAsAtomicUnit=on
  s_rel : Outport
  v_rel : Outport  Port=2
  a_rel : Outport  Port=3
  wires:
  S_rel/1 -> MATLAB Function2/3(Y)
  measurement update/1(X1) -> MATLAB Function2/1(X1)
  MATLAB Function2/1(X2) -> Demux3/1, Delay1/1
  Constant/1 -> time update/1(Q)
  initial_value/1 -> Delay1/3
  Delay/1 -> time update/3(M1)
  time update/2(M2) -> Delay/1
  Delay1/1 -> measurement update/1(X2)
  Constant1/1 -> time update/2(R)
  time update/1(K) -> MATLAB Function2/2(K)
  Demux3/1 -> s_rel/1
  Demux3/2 -> v_rel/1
  Demux3/3 -> a_rel/1
  Jerk/1 -> measurement update/2(u)
  cut_in_flg/1 -> Delay1/2

== system acc_with_sensor/cmd_limiter1/rate_limit ==
  input_raw : Inport
  Sample_Time : Inport  Port=2
  ratelimt_incps : Inport  Port=3
  ratelimt_decps : Inport  Port=4
  Add : Sum  Inputs=+-
  Add1 : Sum
  Constant : Constant  Value=0  SampleTime=T
  Max : MinMax  Function=max  Inputs=2
  Max1 : MinMax  Inputs=2
  Max2 : MinMax  Function=max  Inputs=2
  Max3 : MinMax  Inputs=2
  Product : Product
  Product1 : Product
  Unit Delay : UnitDelay  SampleTime=T  HasFrameUpgradeWarning=on
  ax_cmd1 : Outport
  wires:
  Product1/1 -> Max2/1
  Product/1 -> Max3/2
  Sample_Time/1 -> Product/1, Product1/2
  ratelimt_incps/1 -> Product1/1
  ratelimt_decps/1 -> Product/2
  Constant/1 -> Max2/2, Max3/1
  Max3/1 -> [Dec]
  Max2/1 -> [Inc]
  Unit Delay/1 -> Add1/2, Add/2
  Add1/1 -> ax_cmd1/1, Unit Delay/1
  Max1/1 -> Add1/1
  [Dec] -> Max/2
  [Inc] -> Max1/1
  Max/1 -> Max1/2
  Add/1 -> Max/1
  input_raw/1 -> Add/1

== system acc_with_sensor/cmd_limiter11/rate_limit ==
  input_raw : Inport
  Sample_Time : Inport  Port=2
  ratelimt_incps : Inport  Port=3
  ratelimt_decps : Inport  Port=4
  Add : Sum  Inputs=+-
  Add1 : Sum
  Constant : Constant  Value=0  SampleTime=T
  Max : MinMax  Function=max  Inputs=2
  Max1 : MinMax  Inputs=2
  Max2 : MinMax  Function=max  Inputs=2
  Max3 : MinMax  Inputs=2
  Product : Product
  Product1 : Product
  Unit Delay : UnitDelay  SampleTime=T  HasFrameUpgradeWarning=on
  ax_cmd1 : Outport
  wires:
  input_raw/1 -> Add/1
  Add/1 -> Max/1
  Max/1 -> Max1/2
  [Inc] -> Max1/1
  [Dec] -> Max/2
  Max1/1 -> Add1/1
  Add1/1 -> Unit Delay/1, ax_cmd1/1
  Unit Delay/1 -> Add/2, Add1/2
  Max2/1 -> [Inc]
  Max3/1 -> [Dec]
  Constant/1 -> Max3/1, Max2/2
  ratelimt_decps/1 -> Product/2
  ratelimt_incps/1 -> Product1/1
  Sample_Time/1 -> Product1/2, Product/1
  Product/1 -> Max3/2
  Product1/1 -> Max2/1

== system acc_with_sensor/cmd_limiter2/rate_limit ==
  input_raw : Inport
  Sample_Time : Inport  Port=2
  ratelimt_incps : Inport  Port=3
  ratelimt_decps : Inport  Port=4
  Add : Sum  Inputs=+-
  Add1 : Sum
  Constant : Constant  Value=0  SampleTime=-1
  Max : MinMax  Function=max  Inputs=2
  Max1 : MinMax  Inputs=2
  Max2 : MinMax  Function=max  Inputs=2
  Max3 : MinMax  Inputs=2
  Product : Product
  Product1 : Product
  Unit Delay : UnitDelay  SampleTime=-1  HasFrameUpgradeWarning=on
  ax_cmd1 : Outport
  wires:
  Product1/1 -> Max2/1
  Product/1 -> Max3/2
  Sample_Time/1 -> Product/1, Product1/2
  ratelimt_incps/1 -> Product1/1
  ratelimt_decps/1 -> Product/2
  Constant/1 -> Max2/2, Max3/1
  Max3/1 -> [Dec]
  Max2/1 -> [Inc]
  Unit Delay/1 -> Add1/2, Add/2
  Add1/1 -> ax_cmd1/1, Unit Delay/1
  Max1/1 -> Add1/1
  [Dec] -> Max/2
  [Inc] -> Max1/1
  Max/1 -> Max1/2
  Add/1 -> Max/1
  input_raw/1 -> Add/1

== system acc_with_sensor/cmd_limiter3/rate_limit ==
  input_raw : Inport
  Sample_Time : Inport  Port=2
  ratelimt_incps : Inport  Port=3
  ratelimt_decps : Inport  Port=4
  Add : Sum  Inputs=+-
  Add1 : Sum
  Constant : Constant  Value=0  SampleTime=T
  Max : MinMax  Function=max  Inputs=2
  Max1 : MinMax  Inputs=2
  Max2 : MinMax  Function=max  Inputs=2
  Max3 : MinMax  Inputs=2
  Product : Product
  Product1 : Product
  Unit Delay : UnitDelay  SampleTime=T  HasFrameUpgradeWarning=on
  ax_cmd1 : Outport
  wires:
  Product1/1 -> Max2/1
  Product/1 -> Max3/2
  Sample_Time/1 -> Product/1, Product1/2
  ratelimt_incps/1 -> Product1/1
  ratelimt_decps/1 -> Product/2
  Constant/1 -> Max2/2, Max3/1
  Max3/1 -> [Dec]
  Max2/1 -> [Inc]
  Unit Delay/1 -> Add1/2, Add/2
  Add1/1 -> ax_cmd1/1, Unit Delay/1
  Max1/1 -> Add1/1
  [Dec] -> Max/2
  [Inc] -> Max1/1
  Max/1 -> Max1/2
  Add/1 -> Max/1
  input_raw/1 -> Add/1

== system acc_with_sensor/cmd_limiter4/rate_limit ==
  input_raw : Inport
  Sample_Time : Inport  Port=2
  ratelimt_incps : Inport  Port=3
  ratelimt_decps : Inport  Port=4
  Add : Sum  Inputs=+-
  Add1 : Sum
  Constant : Constant  Value=0  SampleTime=T
  Max : MinMax  Function=max  Inputs=2
  Max1 : MinMax  Inputs=2
  Max2 : MinMax  Function=max  Inputs=2
  Max3 : MinMax  Inputs=2
  Product : Product
  Product1 : Product
  Unit Delay : UnitDelay  SampleTime=T  HasFrameUpgradeWarning=on
  ax_cmd1 : Outport
  wires:
  input_raw/1 -> Add/1
  Add/1 -> Max/1
  Max/1 -> Max1/2
  [Inc] -> Max1/1
  [Dec] -> Max/2
  Max1/1 -> Add1/1
  Add1/1 -> Unit Delay/1, ax_cmd1/1
  Unit Delay/1 -> Add/2, Add1/2
  Max2/1 -> [Inc]
  Max3/1 -> [Dec]
  Constant/1 -> Max3/1, Max2/2
  ratelimt_decps/1 -> Product/2
  ratelimt_incps/1 -> Product1/1
  Sample_Time/1 -> Product1/2, Product/1
  Product/1 -> Max3/2
  Product1/1 -> Max2/1

== system acc_with_sensor/cmd_limiter9/rate_limit ==
  input_raw : Inport
  Sample_Time : Inport  Port=2
  ratelimt_incps : Inport  Port=3
  ratelimt_decps : Inport  Port=4
  Add : Sum  Inputs=+-
  Add1 : Sum
  Constant : Constant  Value=0  SampleTime=T
  Max : MinMax  Function=max  Inputs=2
  Max1 : MinMax  Inputs=2
  Max2 : MinMax  Function=max  Inputs=2
  Max3 : MinMax  Inputs=2
  Product : Product
  Product1 : Product
  Unit Delay : UnitDelay  SampleTime=T  HasFrameUpgradeWarning=on
  ax_cmd1 : Outport
  wires:
  input_raw/1 -> Add/1
  Add/1 -> Max/1
  Max/1 -> Max1/2
  [Inc] -> Max1/1
  [Dec] -> Max/2
  Max1/1 -> Add1/1
  Add1/1 -> Unit Delay/1, ax_cmd1/1
  Unit Delay/1 -> Add/2, Add1/2
  Max2/1 -> [Inc]
  Max3/1 -> [Dec]
  Constant/1 -> Max3/1, Max2/2
  ratelimt_decps/1 -> Product/2
  ratelimt_incps/1 -> Product1/1
  Sample_Time/1 -> Product1/2, Product/1
  Product/1 -> Max3/2
  Product1/1 -> Max2/1

== system acc_with_sensor/Camera/Subsystem6/Subsystem16 ==
  C0 : Inport
  C1 : Inport  Port=2
  "C2 " : Inport  Port=3
  C3 : Inport  Port=4
  VehSpd_mps : Inport  Port=5
  Ax_HV_mps2 : Inport  Port=6
  Add30 : Sum  Inputs=++++
  Add5 : Sum
  Constant10 : Constant  Value=[1:10]'  SampleTime=T
  Constant11 : Constant  Value=0.1  SampleTime=T
  Fcn : Fcn  Expr=(u)^3
  Gain : Gain  Gain=0.5
  Product{,1..2,10..12} (6 alike) : Product
  Square : Math  Operator=square  SignedPower=on  RndMeth=Zero  SaturateOnIntegerOverflow=on
  Square1 : Math  Operator=square  SaturateOnIntegerOverflow=on
  LeftDis : Outport  VectorParamsAs1DForOutWhenUnconnected=off
  wires:
  Constant11/1 -> Product11/2
  VehSpd_mps/1 -> Product10/1
  Add5/1 -> [PrediDis]
  Square1/1 -> Product12/1
  Ax_HV_mps2/1 -> Gain/1
  Product12/1 -> Add5/2
  Product10/1 -> Add5/1
  Gain/1 -> Product12/2
  Product11/1 -> Square1/1, Product10/2
  Constant10/1 -> Product11/1
  C3/1 -> Product2/1
  Add30/1 -> LeftDis/1
  C1/1 -> Product/1
  Product2/1 -> Add30/4
  C0/1 -> Add30/1
  Square/1 -> Product1/2
  Fcn/1 -> Product2/2
  [PrediDis] -> Fcn/1
  [PrediDis] -> Product/2
  "C2 "/1 -> Product1/1
  Product1/1 -> Add30/3
  Product/1 -> Add30/2
  [PrediDis] -> Square/1
